simulink model "mpc_implicito1"  (R2021b)
settings: Solver=VariableStepAuto  StartTime=0.0  StopTime=5933333  FixedStep=1e-3  RelTol=1e-3
undefined symbols (not defined in the file or in its folder): xc7vx485tffg1157
libraries: hdlBasic x137, vmcUtilities x1
settings Model: Creator=fabus  LastModifiedBy=fabus

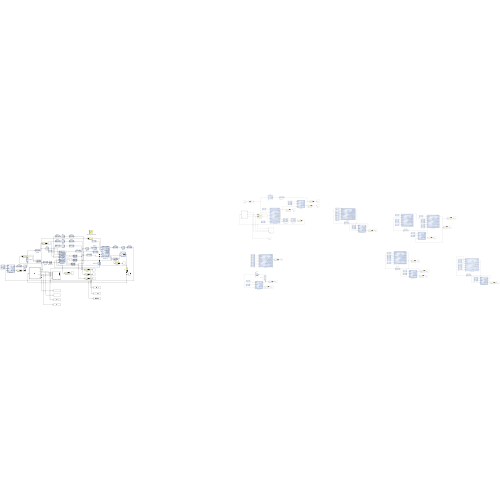
[thumbnail: Simulink's stored preview of the top-level diagram]
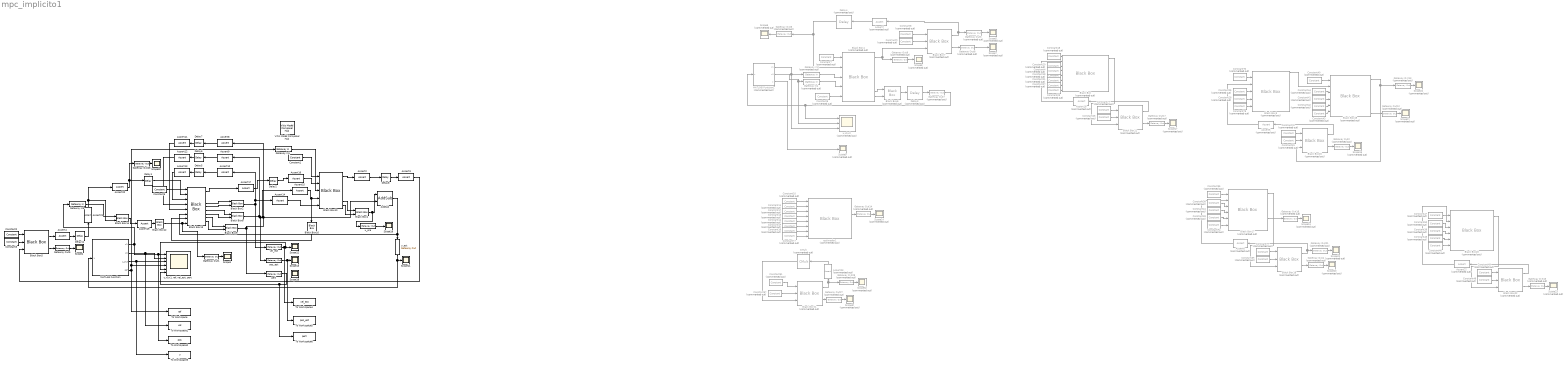
== system mpc_implicito1 ==
  AddSub : hdlBasic/AddSub  mode=Subtraction  use_carryin=off  use_carryout=off  en=off  latency=1  precision=User Defined  arith_type="Signed  (2's comp)"  n_bits=32  bin_pt=fr_width  quantization="Round  (unbiased: +/- Inf)"  overflow=Saturate  use_behavioral_HDL=off  hw_selection=Fabric  pipelined=off  XmcBlockStatus=1  maskContainerNames=tabcontainer1  block_type=addsub  block_config=sysgen:Addsub_config
  Assert{1,5..6,18,22..23} (6 alike) : hdlBasic/Assert  Commented=on  assert_type=off  type_source=Explicitly  gui_display_data_type=Fixed-point  arith_type=Signed (2's comp)  n_bits=16  bin_pt=14  preci_type=Single  exp_width=8  frac_width=24  assert_rate=on  rate_source=Explicitly  period=1  output_port=on  XmcBlockStatus=1  maskContainerNames=group1  block_type=assert  block_config=sysgen:assert_config  block_width=609  block_height=900
  Assert{2..4,8..17,19..21} (16 alike) : hdlBasic/Assert  assert_type=off  type_source=Explicitly  gui_display_data_type=Fixed-point  arith_type=Signed (2's comp)  n_bits=16  bin_pt=14  preci_type=Single  exp_width=8  frac_width=24  assert_rate=on  rate_source=Explicitly  period=1  output_port=on  XmcBlockStatus=1  maskContainerNames=group1  block_type=assert  block_config=sysgen:assert_config  block_width=609  block_height=900
  Black Box : hdlBasic/Black Box  Commented=on  init_code=estimador_func_config  sim_method=Vivado Simulator  verbose=off  XmcBlockStatus=1  maskContainerNames=group1  block_type=blackbox2  block_config=sysgen:black_box_config
  Black Box{1..2,8..9,14} (5 alike) : hdlBasic/Black Box  init_code=valid_out_config  sim_method=Vivado Simulator  verbose=off  XmcBlockStatus=1  maskContainerNames=group1  block_type=blackbox2  block_config=sysgen:black_box_config
  Black Box10 : hdlBasic/Black Box  init_code=mpc_config  sim_method=Vivado Simulator  verbose=off  XmcBlockStatus=1  maskContainerNames=group1  block_type=blackbox2  block_config=sysgen:black_box_config
  Black Box{7,11,15,18,21..22} (6 alike) : hdlBasic/Black Box  Commented=on  init_code=period_setter_config  sim_method=Vivado Simulator  verbose=off  XmcBlockStatus=1  maskContainerNames=group1  block_type=blackbox2  block_config=sysgen:black_box_config
  Black Box12 : hdlBasic/Black Box  init_code=conv_21_to_32_config  sim_method=Vivado Simulator  verbose=off  XmcBlockStatus=1  maskContainerNames=group1  block_type=blackbox2  block_config=sysgen:black_box_config
  Black Box13 : hdlBasic/Black Box  init_code=estimador_func_config  sim_method=Vivado Simulator  verbose=off  XmcBlockStatus=1  maskContainerNames=group1  block_type=blackbox2  block_config=sysgen:black_box_config
  Black Box16 : hdlBasic/Black Box  init_code=conv_21_to_32_config  sim_method=Vivado Simulator  verbose=off  XmcBlockStatus=1  maskContainerNames=group1  block_type=blackbox2  block_config=sysgen:black_box_config
  Black Box17 : hdlBasic/Black Box  Commented=on  init_code=motor_main_config  sim_method=Vivado Simulator  verbose=off  XmcBlockStatus=1  maskContainerNames=group1  block_type=blackbox2  block_config=sysgen:black_box_config
  Black Box19 : hdlBasic/Black Box  Commented=on  init_code=motor_main_config  sim_method=Vivado Simulator  verbose=off  XmcBlockStatus=1  maskContainerNames=group1  block_type=blackbox2  block_config=sysgen:black_box_config
  Black Box20 : hdlBasic/Black Box  Commented=on  init_code=motor_config  sim_method=Vivado Simulator  verbose=off  XmcBlockStatus=1  maskContainerNames=group1  block_type=blackbox2  block_config=sysgen:black_box_config
  Black Box3 : hdlBasic/Black Box  Commented=on  init_code=mpc_config  sim_method=Vivado Simulator  verbose=off  XmcBlockStatus=1  maskContainerNames=group1  block_type=blackbox2  block_config=sysgen:black_box_config
  Black Box4 : hdlBasic/Black Box  Commented=on  init_code=mpc_config  sim_method=Vivado Simulator  verbose=off  XmcBlockStatus=1  maskContainerNames=group1  block_type=blackbox2  block_config=sysgen:black_box_config
  Black Box5 : hdlBasic/Black Box  init_code=period_setter_config  sim_method=Vivado Simulator  verbose=off  XmcBlockStatus=1  maskContainerNames=group1  block_type=blackbox2  block_config=sysgen:black_box_config
  Black Box6 : hdlBasic/Black Box  Commented=on  init_code=valid_out_config  sim_method=Vivado Simulator  verbose=off  XmcBlockStatus=1  maskContainerNames=group1  block_type=blackbox2  block_config=sysgen:black_box_config
  CMult : hdlBasic/CMult  Commented=on  const=1  gui_display_data_type=Fixed-point  const_n_bits=1  const_bin_pt=0  float_type=Single  exp_bits=8  fraction_bits=24  en=off  latency=6  precision=User Defined  arith_type=Unsigned  n_bits=1  bin_pt=0  quantization=Truncate  overflow=Saturate  use_behavioral_HDL=off  mem_type=Distributed RAM  pipeline=off  XmcBlockStatus=1  maskContainerNames=tabcontainer1  block_type=cmult  block_config=sysgen:CMult_config
      settings: infoedit=[]
  Constant1 : hdlBasic/Constant  const=0  gui_display_data_type=Fixed-point  arith_type=Unsigned  n_bits=1  bin_pt=0  preci_type=Single  exp_width=8  frac_width=24  explicit_period=off  period=1  XmcBlockStatus=1  maskContainerNames=tabcontainer1  block_type=constant  block_config=sysgen:Constant_config
  Constant{10,18,27,30,32,35,37,40,47,49} (10 alike) : hdlBasic/Constant  Commented=on  const=0  gui_display_data_type=Fixed-point  arith_type=Unsigned  n_bits=1  bin_pt=0  preci_type=Single  exp_width=8  frac_width=24  explicit_period=on  period=1  XmcBlockStatus=1  maskContainerNames=tabcontainer1  block_type=constant  block_config=sysgen:Constant_config
  Constant11 : hdlBasic/Constant  Commented=on  const=1  gui_display_data_type=Fixed-point  arith_type=Unsigned  n_bits=1  bin_pt=0  preci_type=Single  exp_width=8  frac_width=24  explicit_period=off  period=1  XmcBlockStatus=1  maskContainerNames=tabcontainer1  block_type=constant  block_config=sysgen:Constant_config
  Constant{12..14,17} (4 alike) : hdlBasic/Constant  Commented=on  const=0  gui_display_data_type=Fixed-point  arith_type=Unsigned  n_bits=32  bin_pt=16  preci_type=Single  exp_width=8  frac_width=24  explicit_period=off  period=1  XmcBlockStatus=1  maskContainerNames=tabcontainer1  block_type=constant  block_config=sysgen:Constant_config
  Constant15 : hdlBasic/Constant  Commented=on  const=10  gui_display_data_type=Fixed-point  arith_type=Unsigned  n_bits=32  bin_pt=16  preci_type=Single  exp_width=8  frac_width=24  explicit_period=off  period=1  XmcBlockStatus=1  maskContainerNames=tabcontainer1  block_type=constant  block_config=sysgen:Constant_config
  Constant16 : hdlBasic/Constant  Commented=on  const=10  gui_display_data_type=Fixed-point  arith_type=Unsigned  n_bits=32  bin_pt=16  preci_type=Single  exp_width=8  frac_width=24  explicit_period=off  period=1  XmcBlockStatus=1  maskContainerNames=tabcontainer1  block_type=constant  block_config=sysgen:Constant_config
  Constant{4,19..20,28..29,33..34,39,41..43,45..46} (13 alike) : hdlBasic/Constant  Commented=on  const=0  gui_display_data_type=Fixed-point  arith_type=Unsigned  n_bits=bits  bin_pt=fr_width  preci_type=Single  exp_width=8  frac_width=24  explicit_period=off  period=1  XmcBlockStatus=1  maskContainerNames=tabcontainer1  block_type=constant  block_config=sysgen:Constant_config
  Constant2 : hdlBasic/Constant  const=0  gui_display_data_type=Fixed-point  arith_type=Unsigned  n_bits=1  bin_pt=0  preci_type=Single  exp_width=8  frac_width=24  explicit_period=off  period=1  XmcBlockStatus=1  maskContainerNames=tabcontainer1  block_type=constant  block_config=sysgen:Constant_config
  Constant21 : hdlBasic/Constant  Commented=on  const=0  gui_display_data_type=Fixed-point  arith_type=Unsigned  n_bits=32  bin_pt=fr_width  preci_type=Single  exp_width=8  frac_width=24  explicit_period=off  period=1  XmcBlockStatus=1  maskContainerNames=tabcontainer1  block_type=constant  block_config=sysgen:Constant_config
  Constant22 : hdlBasic/Constant  Commented=on  const=0  gui_display_data_type=Fixed-point  arith_type=Unsigned  n_bits=32  bin_pt=14  preci_type=Single  exp_width=8  frac_width=24  explicit_period=off  period=1  XmcBlockStatus=1  maskContainerNames=tabcontainer1  block_type=constant  block_config=sysgen:Constant_config
  Constant23 : hdlBasic/Constant  Commented=on  const=0  gui_display_data_type=Fixed-point  arith_type=Unsigned  n_bits=32  bin_pt=14  preci_type=Single  exp_width=8  frac_width=24  explicit_period=off  period=1  XmcBlockStatus=1  maskContainerNames=tabcontainer1  block_type=constant  block_config=sysgen:Constant_config
  Constant24 : hdlBasic/Constant  Commented=on  const=-2  gui_display_data_type=Fixed-point  arith_type=Signed (2's comp)  n_bits=bits  bin_pt=fr_width  preci_type=Single  exp_width=8  frac_width=24  explicit_period=off  period=1  XmcBlockStatus=1  maskContainerNames=tabcontainer1  block_type=constant  block_config=sysgen:Constant_config
  Constant25 : hdlBasic/Constant  Commented=on  const=0  gui_display_data_type=Fixed-point  arith_type=Unsigned  n_bits=32  bin_pt=fr_width  preci_type=Single  exp_width=8  frac_width=24  explicit_period=off  period=1  XmcBlockStatus=1  maskContainerNames=tabcontainer1  block_type=constant  block_config=sysgen:Constant_config
  Constant26 : hdlBasic/Constant  Commented=on  const=100  gui_display_data_type=Fixed-point  arith_type=Unsigned  n_bits=32  bin_pt=0  preci_type=Single  exp_width=8  frac_width=24  explicit_period=off  period=1  XmcBlockStatus=1  maskContainerNames=tabcontainer1  block_type=constant  block_config=sysgen:Constant_config
  Constant3 : hdlBasic/Constant  const=1780  gui_display_data_type=Fixed-point  arith_type=Unsigned  n_bits=32  bin_pt=0  preci_type=Single  exp_width=8  frac_width=24  explicit_period=off  period=1  XmcBlockStatus=1  maskContainerNames=tabcontainer1  block_type=constant  block_config=sysgen:Constant_config
  Constant31 : hdlBasic/Constant  Commented=on  const=100  gui_display_data_type=Fixed-point  arith_type=Unsigned  n_bits=32  bin_pt=0  preci_type=Single  exp_width=8  frac_width=24  explicit_period=off  period=1  XmcBlockStatus=1  maskContainerNames=tabcontainer1  block_type=constant  block_config=sysgen:Constant_config
  Constant36 : hdlBasic/Constant  Commented=on  const=103  gui_display_data_type=Fixed-point  arith_type=Unsigned  n_bits=32  bin_pt=0  preci_type=Single  exp_width=8  frac_width=24  explicit_period=off  period=1  XmcBlockStatus=1  maskContainerNames=tabcontainer1  block_type=constant  block_config=sysgen:Constant_config
  Constant38 : hdlBasic/Constant  Commented=on  const=1  gui_display_data_type=Fixed-point  arith_type=Unsigned  n_bits=1  bin_pt=0  preci_type=Single  exp_width=8  frac_width=24  explicit_period=on  period=1  XmcBlockStatus=1  maskContainerNames=tabcontainer1  block_type=constant  block_config=sysgen:Constant_config
  Constant44 : hdlBasic/Constant  Commented=on  const=1  gui_display_data_type=Fixed-point  arith_type=Unsigned  n_bits=1  bin_pt=0  preci_type=Single  exp_width=8  frac_width=24  explicit_period=on  period=1  XmcBlockStatus=1  maskContainerNames=tabcontainer1  block_type=constant  block_config=sysgen:Constant_config
  Constant48 : hdlBasic/Constant  Commented=on  const=301  gui_display_data_type=Fixed-point  arith_type=Unsigned  n_bits=32  bin_pt=0  preci_type=Single  exp_width=8  frac_width=24  explicit_period=off  period=1  XmcBlockStatus=1  maskContainerNames=tabcontainer1  block_type=constant  block_config=sysgen:Constant_config
  Constant5 : hdlBasic/Constant  const=0  gui_display_data_type=Fixed-point  arith_type=Unsigned  n_bits=1  bin_pt=0  preci_type=Single  exp_width=8  frac_width=24  explicit_period=off  period=1  XmcBlockStatus=1  maskContainerNames=tabcontainer1  block_type=constant  block_config=sysgen:Constant_config
  Constant50 : hdlBasic/Constant  Commented=on  const=1  gui_display_data_type=Fixed-point  arith_type=Unsigned  n_bits=1  bin_pt=0  preci_type=Single  exp_width=8  frac_width=24  explicit_period=on  period=1  XmcBlockStatus=1  maskContainerNames=tabcontainer1  block_type=constant  block_config=sysgen:Constant_config
  Constant51 : hdlBasic/Constant  Commented=on  const=0  gui_display_data_type=Fixed-point  arith_type=Unsigned  n_bits=1  bin_pt=0  preci_type=Single  exp_width=8  frac_width=24  explicit_period=off  period=1  XmcBlockStatus=1  maskContainerNames=tabcontainer1  block_type=constant  block_config=sysgen:Constant_config
  Constant52 : hdlBasic/Constant  Commented=on  const=9  gui_display_data_type=Fixed-point  arith_type=Unsigned  n_bits=32  bin_pt=0  preci_type=Single  exp_width=8  frac_width=24  explicit_period=off  period=1  XmcBlockStatus=1  maskContainerNames=tabcontainer1  block_type=constant  block_config=sysgen:Constant_config
  Constant6 : hdlBasic/Constant  Commented=on  const=10  gui_display_data_type=Fixed-point  arith_type=Unsigned  n_bits=32  bin_pt=0  preci_type=Single  exp_width=8  frac_width=24  explicit_period=off  period=1  XmcBlockStatus=1  maskContainerNames=tabcontainer1  block_type=constant  block_config=sysgen:Constant_config
  Constant7 : hdlBasic/Constant  Commented=on  const=0  gui_display_data_type=Fixed-point  arith_type=Unsigned  n_bits=1  bin_pt=0  preci_type=Single  exp_width=8  frac_width=24  explicit_period=off  period=1  XmcBlockStatus=1  maskContainerNames=tabcontainer1  block_type=constant  block_config=sysgen:Constant_config
  Constant8 : hdlBasic/Constant  Commented=on  const=0  gui_display_data_type=Fixed-point  arith_type=Unsigned  n_bits=1  bin_pt=0  preci_type=Single  exp_width=8  frac_width=24  explicit_period=off  period=1  XmcBlockStatus=1  maskContainerNames=tabcontainer1  block_type=constant  block_config=sysgen:Constant_config
  Constant9 : hdlBasic/Constant  Commented=on  const=2400  gui_display_data_type=Fixed-point  arith_type=Unsigned  n_bits=32  bin_pt=0  preci_type=Single  exp_width=8  frac_width=24  explicit_period=on  period=1  XmcBlockStatus=1  maskContainerNames=tabcontainer1  block_type=constant  block_config=sysgen:Constant_config
  Delay{1..2,5..8,11} (7 alike) : hdlBasic/Delay  rst=off  en=off  latency=1  reg_retiming=off  XmcBlockStatus=1  maskContainerNames=group1  block_type=delay  block_config=sysgen:Delay_config
  Delay3 : hdlBasic/Delay  Commented=on  rst=off  en=off  latency=1  reg_retiming=off  XmcBlockStatus=1  maskContainerNames=group1  block_type=delay  block_config=sysgen:Delay_config
  Delay4 : hdlBasic/Delay  Commented=on  rst=off  en=off  latency=1  reg_retiming=off  XmcBlockStatus=1  maskContainerNames=group1  block_type=delay  block_config=sysgen:Delay_config
  Gateway In1 : hdlBasic/Gateway In  gui_display_data_type=Fixed-point  arith_type=Signed (2's comp)  n_bits=32  bin_pt=fr_width  preci_type=Single  exp_width=8  frac_width=24  rows=1  columns=1  quantization="Round  (unbiased: +/- Inf)"  overflow=Saturate  period=1  UseAsADC=off  ADCChannel='1'  interface=None  automatic_assignment=on  address_offset=hex2dec('00')  intf_name=''  intf_description=''  default_value=0  timing_constraint=None  locs_specified=off  LOCs={}  io_standard={}  inherit_from_input=off  hdl_port=on  XmcBlockStatus=1  maskContainerNames=group4  block_type=gatewayin  block_config=sysgen:gateway_in_config  block_width_w=590  block_height_w=620  block_width=640  block_height=850
  Gateway In3 : hdlBasic/Gateway In  Commented=on  gui_display_data_type=Fixed-point  arith_type=Signed (2's comp)  n_bits=32  bin_pt=16  preci_type=Single  exp_width=8  frac_width=24  rows=1  columns=1  quantization="Round  (unbiased: +/- Inf)"  overflow=Saturate  period=1  UseAsADC=off  ADCChannel='1'  interface=None  automatic_assignment=on  address_offset=hex2dec('00')  intf_name=''  intf_description=''  default_value=0  timing_constraint=None  locs_specified=off  LOCs={}  io_standard={}  inherit_from_input=off  hdl_port=on  XmcBlockStatus=1  maskContainerNames=group4  block_type=gatewayin  block_config=sysgen:gateway_in_config  block_width_w=590  block_height_w=620  block_width=640  block_height=850
  Gateway In4 : hdlBasic/Gateway In  Commented=on  gui_display_data_type=Fixed-point  arith_type=Signed (2's comp)  n_bits=32  bin_pt=16  preci_type=Single  exp_width=8  frac_width=24  rows=1  columns=1  quantization="Round  (unbiased: +/- Inf)"  overflow=Saturate  period=1  UseAsADC=off  ADCChannel='1'  interface=None  automatic_assignment=on  address_offset=hex2dec('00')  intf_name=''  intf_description=''  default_value=0  timing_constraint=None  locs_specified=off  LOCs={}  io_standard={}  inherit_from_input=off  hdl_port=on  XmcBlockStatus=1  maskContainerNames=group4  block_type=gatewayin  block_config=sysgen:gateway_in_config  block_width_w=590  block_height_w=620  block_width=640  block_height=850
  Gateway In5 : hdlBasic/Gateway In  gui_display_data_type=Fixed-point  arith_type=Signed (2's comp)  n_bits=W  bin_pt=fr_width  preci_type=Single  exp_width=8  frac_width=24  rows=1  columns=1  quantization=Truncate  overflow=Saturate  period=1  UseAsADC=off  ADCChannel='1'  interface=None  automatic_assignment=on  address_offset=hex2dec('00')  intf_name=''  intf_description=''  default_value=0  timing_constraint=None  locs_specified=off  LOCs={}  io_standard={}  inherit_from_input=off  hdl_port=on  XmcBlockStatus=1  maskContainerNames=group4  block_type=gatewayin  block_config=sysgen:gateway_in_config  block_width_w=590  block_height_w=620  block_width=640  block_height=850
  Gateway Out1 : hdlBasic/Gateway Out  inherit_from_input=off  hdl_port=on  rows=1  columns=1  UseAsDAC=off  DACChannel='1'  interface=None  automatic_assignment=on  address_offset=hex2dec('00')  intf_name=''  intf_description=''  timing_constraint=None  locs_specified=off  LOCs={}  io_standard={}  XmcBlockStatus=1  maskContainerNames=group4  block_type=gatewayout  block_config=sysgen:gateway_out_config  block_width_w=590  block_height_w=620  block_width=620  block_height=750
  Gateway Out{2..4,6..9,12..17,21,27..28} (16 alike) : hdlBasic/Gateway Out  Commented=on  inherit_from_input=off  hdl_port=on  rows=1  columns=1  UseAsDAC=off  DACChannel='1'  interface=None  automatic_assignment=on  address_offset=hex2dec('00')  intf_name=''  intf_description=''  timing_constraint=None  locs_specified=off  LOCs={}  io_standard={}  XmcBlockStatus=1  maskContainerNames=group4  block_type=gatewayout  block_config=sysgen:gateway_out_config  block_width_w=590  block_height_w=620  block_width=620  block_height=750
  Gateway Out26 : hdlBasic/Gateway Out  inherit_from_input=off  hdl_port=on  rows=1  columns=1  UseAsDAC=off  DACChannel='1'  interface=None  automatic_assignment=on  address_offset=hex2dec('00')  intf_name=''  intf_description=''  timing_constraint=None  locs_specified=off  LOCs={}  io_standard={}  XmcBlockStatus=1  maskContainerNames=group4  block_type=gatewayout  block_config=sysgen:gateway_out_config  block_width_w=590  block_height_w=620  block_width=620  block_height=750
  Gateway Out5 : hdlBasic/Gateway Out  inherit_from_input=off  hdl_port=on  rows=1  columns=1  UseAsDAC=off  DACChannel='1'  interface=None  automatic_assignment=on  address_offset=hex2dec('00')  intf_name=''  intf_description=''  timing_constraint=None  locs_specified=off  LOCs={}  io_standard={}  XmcBlockStatus=1  maskContainerNames=group4  block_type=gatewayout  block_config=sysgen:gateway_out_config  block_width_w=590  block_height_w=620  block_width=620  block_height=750
  MATLAB Function : MATLAB Function  TreatAsAtomicUnit=on
  MATLAB Function1 : MATLAB Function  Commented=on  TreatAsAtomicUnit=on
  Scope{1,4,11..13,18..19,30} (8 alike) : Scope
  Scope{5..9,14..15,17,20..25,31..32} (16 alike) : Scope  Commented=on
  To Workspace : ToWorkspace  VariableName=ref  SampleTime=-1
  To Workspace1 : ToWorkspace  VariableName=vel  SampleTime=-1
  To Workspace2 : ToWorkspace  VariableName=pos  SampleTime=-1
  To Workspace3 : ToWorkspace  VariableName=u  SampleTime=-1
  To Workspace4 : ToWorkspace  VariableName=vel_est  SampleTime=-1
  To Workspace5 : ToWorkspace  VariableName=pos_est  SampleTime=-1
  To Workspace6 : ToWorkspace  VariableName=pert  SampleTime=-1
  Vitis Model Composer Hub : vmcUtilities/Vitis Model Composer Hub  Tag=genX  CodeGeneration=off  TargetDirectory=./code  ExportType=AI Engines  IpVendor=xilinx.com  IpLibrary=hls  IpVersion=1.0  IpHWLanguage=Verilog  AieCompilerOptions={}  CreateTestbench=off  TestbenchStackSize=10  RunAieSim=off  AieSimTimeout=50000  RunAieSimProfiling=off  LaunchVitisAnalyzer=off  PlotOutput=off  RunX86Sim=off  X86SimTimeout=10  GenHwImage=off  PlatformType=Not Specified  HwSystemType=Baremetal  HwValidationTarget=hw  ProjDevice=xc7vx485tffg1157-3  ProjDevicePart=xc7vx485tffg1157-3  SamplePeriod=-1  ClockFrequency=200  DataPathParallelism=1  xilinxfamily=virtex7  part=xc7vx485t  speed=-3  package=ffg1157  directory=./netlist  testbench=off  incr_netlist=off  synthesis_tool=Vivado  clock_wrapper=Clock Enables  dbl_ovrd=According to Block Masks  dcm_input_clock_period=10  sysclk_period=10  simulink_period=1  eval_field=0
  estimador1 : hdlBasic/Black Box  Commented=on  init_code=estimador_func_config  sim_method=Vivado Simulator  verbose=off  XmcBlockStatus=1  maskContainerNames=group1  block_type=blackbox2  block_config=sysgen:black_box_config
  pert : hdlBasic/Gateway Out  inherit_from_input=off  hdl_port=on  rows=1  columns=1  UseAsDAC=off  DACChannel='1'  interface=None  automatic_assignment=on  address_offset=hex2dec('00')  intf_name=''  intf_description=''  timing_constraint=None  locs_specified=off  LOCs={}  io_standard={}  XmcBlockStatus=1  maskContainerNames=group4  block_type=gatewayout  block_config=sysgen:gateway_out_config  block_width_w=590  block_height_w=620  block_width=620  block_height=750
  pos_est : hdlBasic/Gateway Out  inherit_from_input=off  hdl_port=on  rows=1  columns=1  UseAsDAC=off  DACChannel='1'  interface=None  automatic_assignment=on  address_offset=hex2dec('00')  intf_name=''  intf_description=''  timing_constraint=None  locs_specified=off  LOCs={}  io_standard={}  XmcBlockStatus=1  maskContainerNames=group4  block_type=gatewayout  block_config=sysgen:gateway_out_config  block_width_w=590  block_height_w=620  block_width=620  block_height=750
  "u,x0,x1, ref, vel_est, pert" : Scope  NumInputPorts=6
  u,x0,x2 : Scope  Commented=on  NumInputPorts=3
  u_act : hdlBasic/Gateway Out  inherit_from_input=off  hdl_port=on  rows=1  columns=1  UseAsDAC=off  DACChannel='1'  interface=None  automatic_assignment=on  address_offset=hex2dec('00')  intf_name=''  intf_description=''  timing_constraint=None  locs_specified=off  LOCs={}  io_standard={}  XmcBlockStatus=1  maskContainerNames=group4  block_type=gatewayout  block_config=sysgen:gateway_out_config  block_width_w=590  block_height_w=620  block_width=620  block_height=750
  u_pre : hdlBasic/Gateway Out  inherit_from_input=off  hdl_port=on  rows=1  columns=1  UseAsDAC=off  DACChannel='1'  interface=None  automatic_assignment=on  address_offset=hex2dec('00')  intf_name=''  intf_description=''  timing_constraint=None  locs_specified=off  LOCs={}  io_standard={}  XmcBlockStatus=1  maskContainerNames=group4  block_type=gatewayout  block_config=sysgen:gateway_out_config  block_width_w=590  block_height_w=620  block_width=620  block_height=750
  vel_est : hdlBasic/Gateway Out  inherit_from_input=off  hdl_port=on  rows=1  columns=1  UseAsDAC=off  DACChannel='1'  interface=None  automatic_assignment=on  address_offset=hex2dec('00')  intf_name=''  intf_description=''  timing_constraint=None  locs_specified=off  LOCs={}  io_standard={}  XmcBlockStatus=1  maskContainerNames=group4  block_type=gatewayout  block_config=sysgen:gateway_out_config  block_width_w=590  block_height_w=620  block_width=620  block_height=750
  wires:
  Constant1/1 -> Black Box10/1
  Black Box2/1 -> Assert10/1, Assert14/1, vel_est/1
  Black Box8/1 -> Assert9/1, pos_est/1, Assert15/1
  Black Box10/8 -> Black Box1/1
  Constant5/1 -> Black Box13/1
  Constant7/1 -> Black Box4/1
  Constant6/1 -> Black Box4/5
  MATLAB Function1/1(x1) -> u,x0,x2/3, Gateway In3/1
  Constant8/1 -> Black Box7/1
  Black Box6/1 -> Delay3/1
  Delay3/1 -> Gateway Out7/1
  Black Box7/1 -> Gateway Out3/1, Assert1/1
  Gateway Out8/1 -> Scope7/1
  Gateway Out3/1 -> Scope5/1
  Gateway In3/1 -> Black Box4/3
  Black Box4/8 -> Black Box6/1
  Constant9/1 -> Black Box7/2
  Black Box4/9 -> Black Box6/2
  MATLAB Function1/3(u) -> Scope9/1
  Black Box7/2 -> Gateway Out8/1
  Assert1/1 -> Delay4/1
  Delay4/1 -> Black Box4/2, Gateway Out6/1
  Gateway Out6/1 -> Scope6/1
  Black Box4/1 -> Gateway Out9/1, Black Box7/3
  Gateway Out7/1 -> u,x0,x2/1, MATLAB Function1/1("u ")
  Gateway In4/1 -> Black Box4/4
  Gateway Out9/1 -> Scope8/1
  MATLAB Function1/2(x0) -> u,x0,x2/2, Gateway In4/1
  Constant2/1 -> Black Box5/1
  Constant3/1 -> Black Box5/2
  Black Box13/9 -> Black Box9/2
  Black Box13/7 -> Black Box8/2
  Black Box13/5 -> Black Box2/2
  Black Box9/1 -> AddSub/2, Assert8/1, pert/1
  Delay5/1 -> Assert13/1
  Delay6/1 -> Assert12/1
  Delay7/1 -> Assert11/1
  Gateway In5/1 -> Black Box14/1
  MATLAB Function/1(x1) -> Gateway In5/1, To Workspace2/1, "u,x0,x1, ref, vel_est, pert"/1
  MATLAB Function/3(u_out) -> To Workspace3/1, "u,x0,x1, ref, vel_est, pert"/3
  MATLAB Function/2(x0) -> To Workspace1/1, "u,x0,x1, ref, vel_est, pert"/2
  Black Box13/1 -> Assert17/1
  Delay2/1 -> Assert16/1
  Black Box5/1 -> Assert4/1
  Gateway Out5/1 -> Scope4/1
  Black Box5/2 -> Gateway Out5/1
  Delay8/1 -> Assert3/1
  Black Box10/1 -> Assert2/1
  Assert2/1 -> Delay8/1
  Assert9/1 -> Delay6/1
  Assert10/1 -> Delay5/1
  Assert11/1 -> Black Box13/5
  Assert12/1 -> Black Box13/4
  Assert17/1 -> Delay2/1
  pos_est/1 -> To Workspace5/1, Scope13/1
  Constant10/1 -> estimador1/1
  Constant11/1 -> estimador1/2
  Constant12/1 -> estimador1/3
  Constant13/1 -> estimador1/4
  Constant14/1 -> estimador1/5
  Constant15/1 -> estimador1/6
  Constant16/1 -> estimador1/7
  Constant17/1 -> estimador1/8
  estimador1/4 -> Gateway Out14/1
  Gateway Out14/1 -> Scope14/1
  Constant20/1 -> Black Box/3
  Constant23/1 -> Black Box/8
  Constant22/1 -> Black Box/7
  Constant21/1 -> Black Box/6
  Black Box11/1 -> Assert18/1
  Constant19/1 -> Black Box/5
  Constant18/1 -> Black Box/1
  Constant4/1 -> Black Box/4
  Constant27/1 -> Black Box11/1
  Constant26/1 -> Black Box11/2
  Black Box/1 -> Black Box11/3
  Gateway Out17/1 -> Scope17/1
  Black Box11/2 -> Gateway Out17/1
  Assert18/1 -> Black Box/2
  Black Box13/8 -> Black Box9/1
  u_act/1 -> MATLAB Function/1(u), Scope11/1
  Gateway Out1/1 -> Scope1/1
  Assert8/1 -> Delay7/1
  Black Box14/1 -> Assert19/1
  Gateway In1/1 -> Black Box10/3
  MATLAB Function/4(ref) -> Gateway In1/1, "u,x0,x1, ref, vel_est, pert"/4, To Workspace/1
  Assert14/1 -> Black Box10/5
  Assert13/1 -> Black Box13/3
  Assert3/1 -> Black Box5/3
  Assert19/1 -> Black Box12/1
  Delay11/1 -> Assert21/1
  Black Box10/9 -> Black Box1/2
  Black Box1/1 -> u_pre/1, AddSub/1
  Assert21/1 -> Assert20/1, Black Box14/2
  Assert20/1 -> Delay1/1, Gateway Out26/1
  Assert4/1 -> Delay11/1
  Delay1/1 -> Black Box13/2
  Assert15/1 -> Black Box10/4, Black Box16/1
  u_pre/1 -> Scope19/1
  Black Box13/4 -> Black Box2/1
  Black Box13/6 -> Black Box8/1
  Assert5/1 -> Black Box3/2
  Constant25/1 -> Black Box3/3
  Constant28/1 -> Black Box3/4
  Constant29/1 -> Black Box3/5
  Constant30/1 -> Black Box3/1
  Gateway Out2/1 -> Scope15/1
  Black Box15/2 -> Gateway Out2/1
  Constant31/1 -> Black Box15/2
  Black Box15/1 -> Assert5/1
  Constant32/1 -> Black Box15/1
  Constant33/1 -> Black Box17/5
  Assert6/1 -> Black Box17/2
  Constant35/1 -> Black Box17/1
  Black Box17/1 -> Black Box18/3
  Constant24/1 -> Black Box17/4
  Constant37/1 -> Black Box18/1
  Black Box18/2 -> Gateway Out4/1
  Gateway Out4/1 -> Scope20/1
  Constant36/1 -> Black Box18/2
  Constant34/1 -> Black Box17/6
  Black Box18/1 -> Gateway Out21/1, Assert6/1
  Constant38/1 -> Black Box17/3
  Black Box3/1 -> Black Box19/2
  Constant40/1 -> Black Box19/1
  Constant41/1 -> Black Box19/4
  Constant44/1 -> Black Box19/3
  Constant42/1 -> Black Box19/5
  Constant43/1 -> Black Box19/6
  Gateway Out12/1 -> Scope21/1
  Black Box19/5 -> Gateway Out12/1
  Gateway Out13/1 -> Scope22/1
  Black Box19/1 -> Gateway Out13/1, Black Box15/3
  Black Box20/1 -> Black Box22/3
  Constant45/1 -> Black Box20/5
  Constant46/1 -> Black Box20/6
  Gateway Out15/1 -> Scope23/1
  Constant49/1 -> Black Box22/1
  Black Box22/1 -> Assert22/1
  Constant48/1 -> Black Box22/2
  Constant47/1 -> Black Box20/1
  Constant50/1 -> Black Box20/3
  Constant39/1 -> Black Box20/4
  Assert22/1 -> Black Box20/2
  Black Box22/2 -> Gateway Out15/1
  Gateway Out16/1 -> Scope24/1
  Black Box17/4 -> Gateway Out16/1
  Gateway Out21/1 -> Scope25/1
  Black Box12/1 -> Gateway Out1/1, Black Box13/8
  Assert16/1 -> Black Box10/2
  Black Box16/1 -> Black Box13/7
  AddSub/1 -> Black Box13/6, u_act/1
  Gateway Out26/1 -> Scope30/1
  Constant52/1 -> Black Box21/2
  Gateway Out27/1 -> Scope31/1
  Black Box21/2 -> Gateway Out27/1
  Constant51/1 -> Black Box21/1
  CMult/1 -> Black Box21/3
  Assert23/1 -> CMult/1
  Gateway Out28/1 -> Scope32/1
  Black Box21/1 -> Gateway Out28/1, Assert23/1
  vel_est/1 -> To Workspace4/1, Scope12/1, "u,x0,x1, ref, vel_est, pert"/5
  pert/1 -> To Workspace6/1, "u,x0,x1, ref, vel_est, pert"/6

== matlab function mpc_implicito1/MATLAB Function1 ==
  data: x1 output; x0 output; u input; u output
function [x1,x0, u] = fcn(u)


    if isnan(u)
        u = 0;
    end
    if abs(u) < 0.03
        u = 0;
    end
    h = 4.17e-8;         % Ts: Periodo de muestreo en segundos
     % Declare a persistent variable
    persistent estado
    %u=0;
    if isempty(estado)
        estado = double([3.0;-1.0]);
    end
    

    %a = 29.4797;
    %K = 45.9744;
    a = 28.8582;
    K = 45.0051;
    %ve d i s c r e t o
    A=[exp(-a*h) 0; (1-exp(-a*h))/a 1 ];
    B=[1-exp(-a*h); exp(-a*h)/a-1/a+h ]*K/a;

    estado = A*estado + B*u;
    
    x0 = estado(1); %vel
    x1 = estado(2); %pos
%     
%

== matlab function mpc_implicito1/MATLAB Function ==
  data: x1 output; x0 output; u input; u_out output; ref output
function [x1,x0, u_out, ref] = fcn(u)
    u_out = u;
    %u = fi(u, 1, 64, 32);
    if isnan(u)
        u = 0;
    end
    if u>10
        u=10;
    end
    if u<-10
        u=-10;
    end
    if abs(u) < 0.3
        u = 0;
    end
    h = (12e-3)/1780;         % Ts: Periodo de muestreo en segundos
     % Declare a persistent variable
    persistent estado
    %u=0;
    if isempty(estado)
        estado = double([0;0]);
    end
    

    %a = 29.4797;
    %K = 45.9744;
    a = 28.8582;
    K = 45.0051;
    %ve d i s c r e t o
    A=[exp(-a*h) 0; (1-exp(-a*h))/a 1 ];
    B=[1-exp(-a*h); exp(-a*h)/a-1/a+h ]*K/a;

    estado = A*estado + B*u;
    
    x0 = estado(1); %vel
    x1 = estado(2); %pos
    
    %referencia
    persistent T
    if isempty(T)
        T = 0;
    end
    T = T+1;
    persistent ref_arriba
    if isempty(ref_arriba)
        ref_arriba = 1;
    end
    if(T > 1780*10/(12e-3))
        T=0;
        if(ref_arriba == 1)
            ref_arriba = 0;
        else
            ref_arriba = 1;
        end
    end

    if(ref_arriba == 1)
        ref = 350*pi/180;
    else
        ref = 10*pi/180;
    end
